simulink model "PID_digital_tarea"  (R2016a)
settings: Solver=ode45  StartTime=0.0  StopTime=7  MaxStep=1e-5  RelTol=1e-3
values from neighbouring files (symbols this model uses):
  c1 = -10    [actividad_2.m]
  K = 10    [actividad_2.m]
  Kd = K * c    [actividad_2.m]
  Ki = simplify(Ki)    [actividad_2.m]
  Kp = simplify(Kp)    [actividad_2.m]
  p1 = -3    [actividad_2.m]
  p2 = -2    [actividad_2.m]
  T = 0.09    [actividad_2.m]
undefined symbols (not defined in the file or in its folder): DiscIntNeverNeededParam
libraries: simulink x1
settings Model: Creator=Usuario  LastModifiedBy=PC
settings DataIOCC: SaveFormat=Array  SignalLoggingSaveFormat=ModelDataLogs
settings OptimizationCC: InitFltsAndDblsToZero=on
settings DebuggingCC: SaveWithParameterizedLinksMsg=none  UnderspecifiedInitializationDetection=Classic  MergeDetectMultiDrivingBlocksExec=none  SignalResolutionControl=TryResolveAllWithWarning  SolverPrmCheckMsg=warning  MultiTaskDSMMsg=warning  MultiTaskCondExecSysMsg=none  FcnCallInpInsideContextMsg=UseLocalSettings
settings HardwareCC: ProdBitPerPointer=32  ProdLargestAtomicFloat=None  ProdIntDivRoundTo=Undefined  ProdEndianess=Unspecified  ProdWordSize=32  ProdHWDeviceType=32-bit Generic
settings ModelReferenceCC: PropagateSignalLabelsOutOfModel=off
settings GRTTargetCC: TargetFcnLib=ansi_tfl_tmw.mat  CombineOutputUpdateFcns=off  GRTInterface=on
settings ConfigComp: CovModelRefEnable=Off  CovSFcnEnable=off

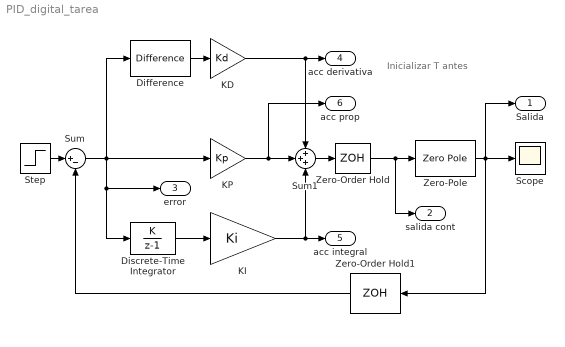
== system PID_digital_tarea ==
  note: Inicializar T antes
  Difference : simulink/Discrete/Difference  ICPrevInput=0.0  InputProcessing=Inherited  OutMin=[]  OutMax=[]  OutDataType=fixdt(1, 16)  OutScaling=2^-10  DoSatur=off
  Discrete-Time Integrator : DiscreteIntegrator  IntegratorMethod=Accumulation: Forward Euler  SampleTime=-1  ICPrevOutput=DiscIntNeverNeededParam  ICPrevScaledInput=DiscIntNeverNeededParam
  KD : Gain  Gain=Kd
  KI : Gain  Gain=Ki
  KP : Gain  Gain=Kp
  Scope : Scope
  Step : Step  Time=0  SampleTime=T
  Sum : Sum  Inputs=|+-
  Sum1 : Sum  Inputs=+++
  Zero-Order Hold : ZeroOrderHold  SampleTime=T
  Zero-Order Hold1 : ZeroOrderHold  SampleTime=T
  Zero-Pole : ZeroPole  Zeros=[c1]  Poles=[p1 p2]  Gain=[K]
  Salida : Outport
  salida cont : Outport  Port=2
  error : Outport  Port=3
  acc derivativa : Outport  Port=4
  acc integral : Outport  Port=5
  acc prop : Outport  Port=6
  wires:
  Zero-Order Hold/1 -> Zero-Pole/1, salida cont/1
  Step/1 -> Sum/1
  Zero-Pole/1 -> Zero-Order Hold1/1, Scope/1, Salida/1
  KI/1 -> Sum1/3, acc integral/1
  KP/1 -> acc prop/1, Sum1/2
  Zero-Order Hold1/1 -> Sum/2
  Sum/1 -> Difference/1, Discrete-Time Integrator/1, error/1, KP/1
  Sum1/1 -> Zero-Order Hold/1
  KD/1 -> Sum1/1, acc derivativa/1
  Difference/1 -> KD/1
  Discrete-Time Integrator/1 -> KI/1
